simulink model "planta_foguete"  (R2024a)
settings: Solver=VariableStepAuto  StartTime=0.0  StopTime=10.0  RelTol=1e-3
values from neighbouring files (symbols this model uses):
  x0_sim = [ic.x0; ic.y0; ic.h0; 0; 0; ic.vz0;                ic.phi0; ic.theta0; 0; 0; ic.q0; 0; ic.m0]    [envelope_mais_monte_carlo_final.m]    (also in init_mpc.m = [p.x0; p.y0; p.h0; init_sim.m = [p.x0)
libraries: simulink_extras x6, simulink x1
settings Model: Creator=marin  LastModifiedBy=marin

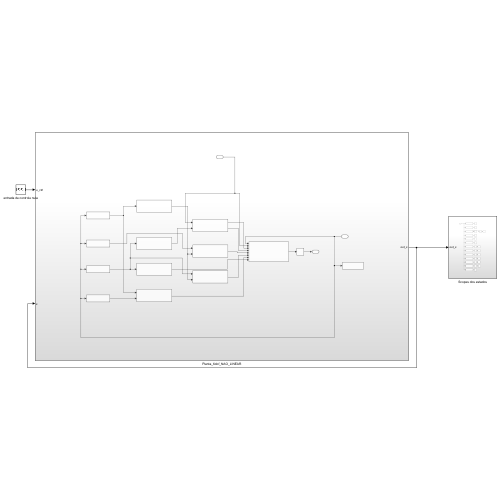
[thumbnail: Simulink's stored preview of the top-level diagram]
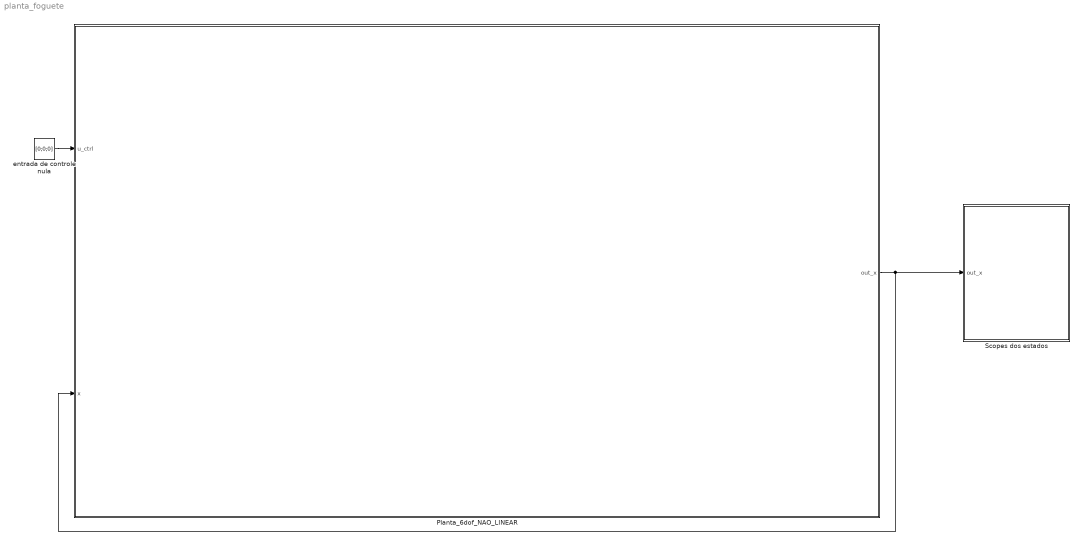
== system planta_foguete ==
  Planta_6dof_NAO_LINEAR : Subsystem
  Scopes dos estados : Subsystem
  entrada de controle nula : Constant  Value=[0;0;0]
  wires:
  Planta_6dof_NAO_LINEAR/1(out_x) -> Scopes dos estados/1(out_x), Planta_6dof_NAO_LINEAR/2(x)
  entrada de controle nula/1 -> Planta_6dof_NAO_LINEAR/1(u_ctrl)

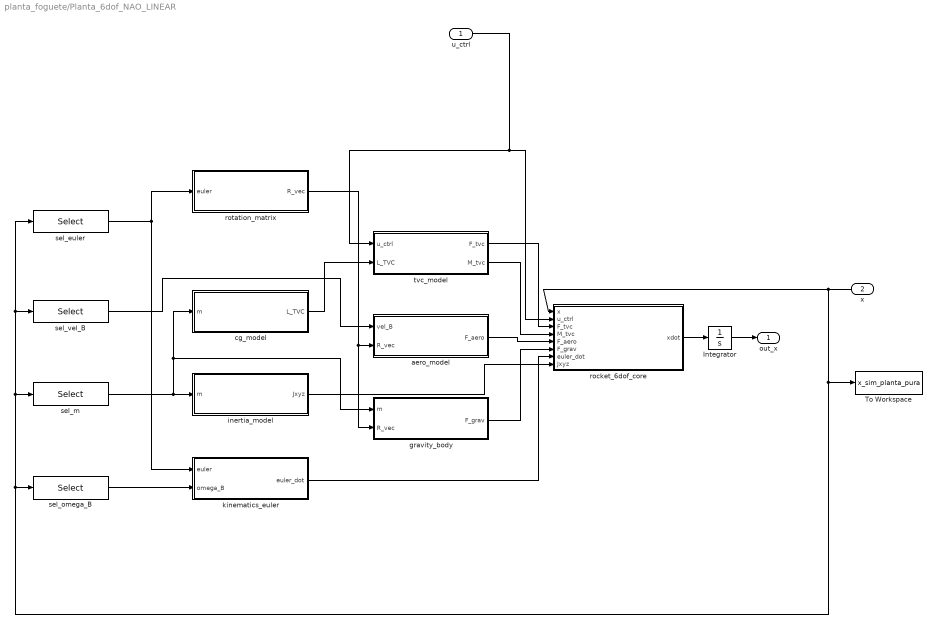
== system planta_foguete/Planta_6dof_NAO_LINEAR ==
  u_ctrl : Inport
  x : Inport  Port=2
  Integrator : Integrator  InitialCondition=x0_sim
  To Workspace : ToWorkspace  VariableName=x_sim_planta_pura  SaveFormat=Timeseries  SampleTime=0.01
  aero_model : MATLAB Function  TreatAsAtomicUnit=on
  cg_model : MATLAB Function  TreatAsAtomicUnit=on
  gravity_body : MATLAB Function  TreatAsAtomicUnit=on
  inertia_model : MATLAB Function  TreatAsAtomicUnit=on
  kinematics_euler : MATLAB Function  TreatAsAtomicUnit=on
  rocket_6dof_core : MATLAB Function  TreatAsAtomicUnit=on
  rotation_matrix : MATLAB Function  TreatAsAtomicUnit=on
  sel_euler : Selector  InputPortWidth=13  IndexOptions=Index vector (dialog)  Indices=7:9  OutputSizes=1
  sel_m : Selector  InputPortWidth=13  IndexOptions=Index vector (dialog)  Indices=13  OutputSizes=1
  sel_omega_B : Selector  InputPortWidth=13  IndexOptions=Index vector (dialog)  Indices=10:12  OutputSizes=1
  sel_vel_B : Selector  InputPortWidth=13  IndexOptions=Index vector (dialog)  Indices=4:6  OutputSizes=1
  tvc_model : MATLAB Function  TreatAsAtomicUnit=on
  out_x : Outport
  wires:
  sel_vel_B/1 -> aero_model/1(vel_B)
  cg_model/1(L_TVC) -> tvc_model/2(L_TVC)
  inertia_model/1(Jxyz) -> rocket_6dof_core/8(Jxyz)
  x/1 -> rocket_6dof_core/1(x), To Workspace/1, sel_m/1, sel_vel_B/1, sel_euler/1, sel_omega_B/1
  sel_m/1 -> cg_model/1(m), gravity_body/1(m), inertia_model/1(m)
  kinematics_euler/1(euler_dot) -> rocket_6dof_core/7(euler_dot)
  gravity_body/1(F_grav) -> rocket_6dof_core/6(F_grav)
  tvc_model/2(M_tvc) -> rocket_6dof_core/4(M_tvc)
  rotation_matrix/1(R_vec) -> gravity_body/2(R_vec), aero_model/2(R_vec)
  aero_model/1(F_aero) -> rocket_6dof_core/5(F_aero)
  u_ctrl/1 -> tvc_model/1(u_ctrl), rocket_6dof_core/2(u_ctrl)
  tvc_model/1(F_tvc) -> rocket_6dof_core/3(F_tvc)
  Integrator/1 -> out_x/1
  rocket_6dof_core/1(xdot) -> Integrator/1
  sel_omega_B/1 -> kinematics_euler/2(omega_B)
  sel_euler/1 -> rotation_matrix/1(euler), kinematics_euler/1(euler)

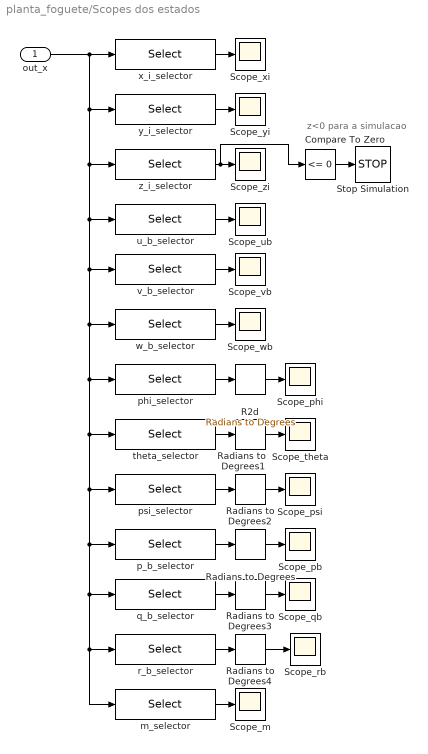
== system planta_foguete/Scopes dos estados ==
  note: z<0 para a simulacao
  out_x : Inport
  Compare To Zero : simulink/Logic and Bit Operations/Compare To Zero  relop=<=  OutDataTypeStr=boolean
  R2d : simulink_extras/Transformations/Radians to Degrees
  Radians to Degrees{,1..4} (5 alike) : simulink_extras/Transformations/Radians to Degrees
  Scope_m : Scope
  Scope_pb : Scope
  Scope_phi : Scope
  Scope_psi : Scope
  Scope_qb : Scope
  Scope_rb : Scope
  Scope_theta : Scope
  Scope_ub : Scope
  Scope_vb : Scope
  Scope_wb : Scope
  Scope_xi : Scope
  Scope_yi : Scope
  Scope_zi : Scope
  Stop Simulation : Stop
  m_selector : Selector  InputPortWidth=13  IndexOptions=Index vector (dialog)  Indices=13  OutputSizes=1
  p_b_selector : Selector  InputPortWidth=13  IndexOptions=Index vector (dialog)  Indices=10  OutputSizes=1
  phi_selector : Selector  InputPortWidth=13  IndexOptions=Index vector (dialog)  Indices=7  OutputSizes=1
  psi_selector : Selector  InputPortWidth=13  IndexOptions=Index vector (dialog)  Indices=9  OutputSizes=1
  q_b_selector : Selector  InputPortWidth=13  IndexOptions=Index vector (dialog)  Indices=11  OutputSizes=1
  r_b_selector : Selector  InputPortWidth=13  IndexOptions=Index vector (dialog)  Indices=12  OutputSizes=1
  theta_selector : Selector  InputPortWidth=13  IndexOptions=Index vector (dialog)  Indices=8  OutputSizes=1
  u_b_selector : Selector  InputPortWidth=13  IndexOptions=Index vector (dialog)  Indices=4  OutputSizes=1
  v_b_selector : Selector  InputPortWidth=13  IndexOptions=Index vector (dialog)  Indices=5  OutputSizes=1
  w_b_selector : Selector  InputPortWidth=13  IndexOptions=Index vector (dialog)  Indices=6  OutputSizes=1
  x_i_selector : Selector  InputPortWidth=13  IndexOptions=Index vector (dialog)  Indices=1  OutputSizes=1
  y_i_selector : Selector  InputPortWidth=13  IndexOptions=Index vector (dialog)  Indices=2  OutputSizes=1
  z_i_selector : Selector  InputPortWidth=13  IndexOptions=Index vector (dialog)  Indices=3  OutputSizes=1
  wires:
  u_b_selector/1 -> Scope_ub/1
  y_i_selector/1 -> Scope_yi/1
  v_b_selector/1 -> Scope_vb/1
  x_i_selector/1 -> Scope_xi/1
  w_b_selector/1 -> Scope_wb/1
  m_selector/1 -> Scope_m/1
  z_i_selector/1 -> Compare To Zero/1, Scope_zi/1
  out_x/1 -> v_b_selector/1, m_selector/1, r_b_selector/1, q_b_selector/1, p_b_selector/1, psi_selector/1, theta_selector/1, phi_selector/1, w_b_selector/1, u_b_selector/1, z_i_selector/1, y_i_selector/1, x_i_selector/1
  Compare To Zero/1 -> Stop Simulation/1
  phi_selector/1 -> R2d/1
  R2d/1 -> Scope_phi/1
  theta_selector/1 -> Radians to Degrees1/1
  Radians to Degrees1/1 -> Scope_theta/1
  psi_selector/1 -> Radians to Degrees2/1
  Radians to Degrees2/1 -> Scope_psi/1
  p_b_selector/1 -> Radians to Degrees/1
  Radians to Degrees/1 -> Scope_pb/1
  q_b_selector/1 -> Radians to Degrees3/1
  Radians to Degrees3/1 -> Scope_qb/1
  Radians to Degrees4/1 -> Scope_rb/1
  r_b_selector/1 -> Radians to Degrees4/1

== matlab function planta_foguete/Planta_6dof_NAO_LINEAR/aero_model ==
  data: vel_B input; F_aero output; R_vec input
function F_aero = fcn(vel_B, R_vec)
% hardcoded aqui no bloco (identico ao .m correspondente),
% para evitar coder.extrinsic, que estava reclamando 
rho = 1.225;  Sref = 10.52;  CD0 = 0.30;

R_IB  = reshape(R_vec, 3, 3);
v_rel = vel_B;   % vento = 0 nominal
v_mag = norm(v_rel);
if v_mag < 1e-6
    F_aero = zeros(3,1);
else
    D      = 0.5 * rho * v_mag^2 * Sref * CD0;
    F_aero = -D * (v_rel / v_mag);
end

== matlab function planta_foguete/Planta_6dof_NAO_LINEAR/cg_model ==
  data: m input; L_TVC output
function L_TVC = fcn(m)
% hardcoded aqui no bloco (identico ao .m correspondente),
% para evitar coder.extrinsic, que estava reclamando 
r_CG_0 = 18.5;   r_CG_f = 17.0;
m0 = 30000;       mf = 22500;

frac  = max(0, min(1, (m - mf) / (m0 - mf)));
L_TVC = r_CG_f + (r_CG_0 - r_CG_f) * frac;

== matlab function planta_foguete/Planta_6dof_NAO_LINEAR/gravity_body ==
  data: m input; F_grav output; R_vec input
function F_grav = fcn(m, R_vec)
g    = 9.80665;
R_IB = reshape(R_vec, 3, 3);
F_grav = m * (R_IB' * [0; 0; -g]);

== matlab function planta_foguete/Planta_6dof_NAO_LINEAR/inertia_model ==
  data: m input; Jxyz output
function Jxyz = fcn(m)
% hardcoded aqui no bloco (identico ao .m correspondente),
% para evitar coder.extrinsic, que estava reclamando 
m0 = 30000;  mf = 22500;
Jzz0 = 8.741e4;  Jzz_f = 7.485e4;
Jxx0 = 3.805e6;  Jxx_f = 3.202e6;

frac = max(0, min(1, (m - mf) / (m0 - mf)));
Jzz  = Jzz_f + (Jzz0 - Jzz_f) * frac;
Jxx  = Jxx_f + (Jxx0 - Jxx_f) * frac;
Jxyz = [Jxx; Jxx; Jzz];  % [Jxx; Jyy=Jxx; Jzz]

== matlab function planta_foguete/Planta_6dof_NAO_LINEAR/kinematics_euler ==
  data: euler input; euler_dot output; omega_B input
function euler_dot = fcn(euler, omega_B)
% Chama kinematics_euler.m
euler_dot = kinematics_euler(euler, omega_B);

== matlab function planta_foguete/Planta_6dof_NAO_LINEAR/rocket_6dof_core ==
  data: x input; xdot output; u_ctrl input; F_tvc input; M_tvc input; F_aero input; F_grav input; euler_dot input; Jxyz input
function xdot = fcn(x, u_ctrl, F_tvc, M_tvc, F_aero, F_grav, euler_dot, Jxyz)
% Montagem final das EDOs 6-DOF. Forças, momentos, euler_dot e inércia
% chegam prontos de blocos a montante; aqui só monta Newton-Euler.
% hardcoded aqui no bloco (identico ao .m correspondente),
% para evitar coder.extrinsic, que estava reclamando
T_max = 845000;  T_min = 338000;
Isp = 282;       g0 = 9.80665;   mf = 22500;
vel_B   = x(4:6);
euler   = x(7:9);
omega_B = x(10:12);
m       = max(mf, x(13));
T       = max(T_min, min(T_max, u_ctrl(1)));
% R_IB
phi=euler(1); theta=euler(2); psi=euler(3);
R_IB = rotation_matrix(phi, theta, psi);
% EQ
pos_dot = R_IB * vel_B;
% EQ
F_total = F_tvc + F_aero + F_grav;
vel_dot = (1/m)*F_total - cross(omega_B, vel_B);   % Coriolis no corpo
% EQ
Jxx=Jxyz(1); Jyy=Jxyz(2); Jzz=Jxyz(3);
J    = diag([Jxx; Jyy; Jzz]);
Jinv = diag([1/Jxx; 1/Jyy; 1/Jzz]);
omega_dot = Jinv*(M_tvc - cross(omega_B, J*omega_B));   % termo giroscopico
% EQ
if x(13) > mf + 1.0    % margem evita oscilar massa em torno de mf
    m_dot = -T/(Isp*g0);
else
    m_dot = 0;
end
xdot = [pos_dot; vel_dot; euler_dot; omega_dot; m_dot];

== matlab function planta_foguete/Planta_6dof_NAO_LINEAR/rotation_matrix ==
  data: euler input; R_vec output
function R_vec = fcn(euler)
% Chama rotation_matrix.m -> achata 3x3 para 9x1
R     = rotation_matrix(euler(1), euler(2), euler(3));
R_vec = R(:);

== matlab function planta_foguete/Planta_6dof_NAO_LINEAR/tvc_model ==
  data: u_ctrl input; F_tvc output; L_TVC input; M_tvc output
function [F_tvc, M_tvc] = fcn(u_ctrl, L_TVC)
% Chama tvc_model.m  |  u_ctrl = [T; delta_y; delta_x]
[F_tvc, M_tvc] = tvc_model(u_ctrl(1), u_ctrl(2), u_ctrl(3), L_TVC);
